simulink model "main"  (R2023b)
settings: Solver=ode4  StartTime=0.0  StopTime=100  FixedStep=0.001  RelTol=1e-3  EnableMultiTasking=on
PreLoadFcn:
  | UserInputs;
libraries: uavalgslib x1, simulink x1
settings Model: DataDictionary=topLevel.sldd  Creator=luke  LastModifiedBy=luke
settings DebuggingCC: InheritedTsInSrcMsg=none
settings ModelReferenceCC: EnableRefExpFcnMdlSchedulingChecks=on  PropagateSignalLabelsOutOfModel=off

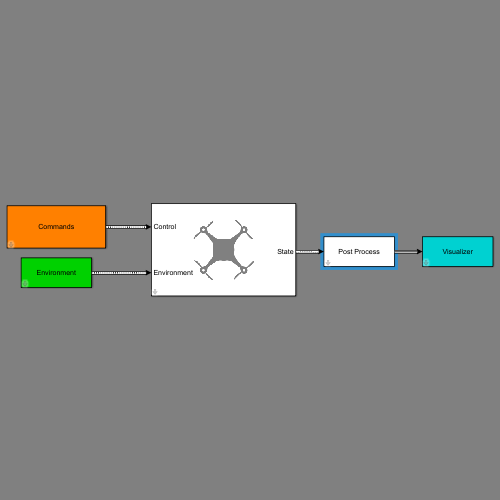
[thumbnail: Simulink's stored preview of the top-level diagram]
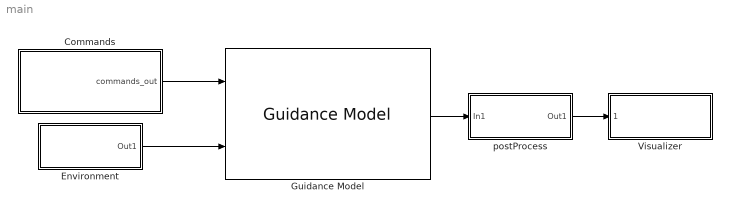
== system main ==
  Commands : Subsystem
      mask Display: disp('Commands');
  Environment : Subsystem
      mask Display: disp('Environment');
  Guidance Model : uavalgslib/Guidance Model  ModelType=MultirotorGuidance  SpecifiedDataType=double  SimulateUsing=Interpreted execution  InitialWorldPositionMultirotor=[0; 0; 200]  InitialWorldVelocityMultirotor=[10; 0; 0]  InitialEulerZYXMultirotor=[0; 0.1; 0]  InitialBodyAngularRateRPYMultirotor=[0; 0; 0]  InitialThrustMultirotor=0  InitialNorthFixedWing=0  InitialEastFixedWing=0  InitialHeightFixedWing=10  InitialAirSpeedFixedWing=0  InitialHeadingAngleFixedWing=0  InitialFlightPathAngleFixedWing=0  InitialRollAngleFixedWing=0  InitialRollAngleRateFixedWing=0  PDRollMultirotor=[3402.97,116.67]  PDPitchMultirotor=[3402.97, 116.67]  PYawRateMultirotor=1950  PThrustMultirotor=3900  MassMultirotor=0.1  PHeightFixedWing=3.9  PHeadingAngleFixedWing=3.9  PFlightPathAngleFixedWing=39  PDRollFixedWing=[3402.97, 116.67]  PAirSpeedFixedWing=1  FlightPathAngleLimitsFixedWing=[-pi/2, pi/2]  StateBusName='StateBus'  ControlBusName='ControlBus'  EnvironmentBusName='EnvironmentBus'  DataType=double
  Visualizer : Subsystem  ReferencedSubsystem=Visualizer
  postProcess : Subsystem
      mask Display: disp("Post Process");
  wires:
  Commands/1(commands_out) -> Guidance Model/1
  Guidance Model/1 -> postProcess/1(In1)
  Environment/1(Out1) -> Guidance Model/2
  postProcess/1(Out1) -> Visualizer/1

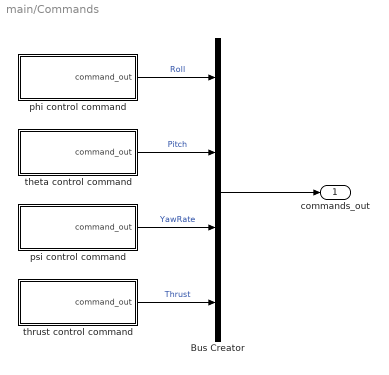
== system main/Commands ==
  Bus Creator : BusCreator  Inputs=4  OutDataTypeStr=Bus: ControlBus  NonVirtualBus=on
      settings: InheritFromInputs=off
  phi control command : Subsystem  Variant=on
      mask Display: disp('\phi Control Command', 'Texmode', 'on');
  psi control command : Subsystem  Variant=on
      mask Display: disp('\psi Control Command', 'Texmode', 'on');
  theta control command : Subsystem  Variant=on
      mask Display: disp('\theta Control Command', 'Texmode', 'on');
  thrust control command : Subsystem  Variant=on
      mask Display: disp('Thrust Control Command');
  commands_out : Outport  OutDataTypeStr=Bus: ControlBus
  wires:
  Bus Creator/1 -> commands_out/1
  theta control command/1(command_out) -> Bus Creator/2  "Pitch"
  phi control command/1(command_out) -> Bus Creator/1  "Roll"
  psi control command/1(command_out) -> Bus Creator/3  "YawRate"
  thrust control command/1(command_out) -> Bus Creator/4  "Thrust"

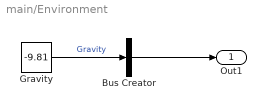
== system main/Environment ==
  Bus Creator : BusCreator  Inputs=1  OutDataTypeStr=Bus: EnvironmentBus  NonVirtualBus=on
      settings: InheritFromInputs=off
  Gravity : Constant  Value=-9.81
  Out1 : Outport  OutDataTypeStr=Bus: EnvironmentBus
  wires:
  Bus Creator/1 -> Out1/1
  Gravity/1 -> Bus Creator/1  "Gravity"

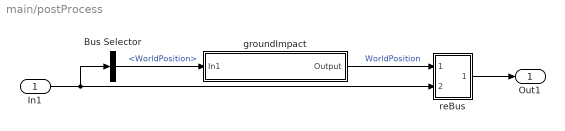
== system main/postProcess ==
  In1 : Inport  OutDataTypeStr=Bus: StateBus
  Bus Selector : BusSelector  OutputSignals=WorldPosition
  groundImpact : Subsystem
      mask Display: disp('Ground Impact');
  reBus : Subsystem
  Out1 : Outport  OutDataTypeStr=Bus: StateBus
  wires:
  reBus/1(Out1) -> Out1/1
  In1/1 -> reBus/2(In1), Bus Selector/1
  groundImpact/1(Output) -> reBus/1(WorldPostion)  "WorldPosition"
  Bus Selector/1 -> groundImpact/1(In1)  "<WorldPosition>"

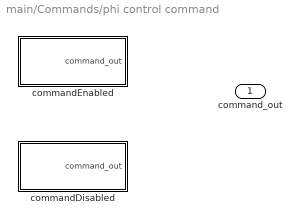
== system main/Commands/phi control command ==
  commandDisabled : Subsystem  VariantControl="userInputs.commands.commandFlags.phiEnable  ==0"
      mask Display: disp('Command Disabled');
  commandEnabled : Subsystem  VariantControl="userInputs.commands.commandFlags.phiEnable  == 1"
      mask Display: disp('Command Enabled');
  command_out : Outport

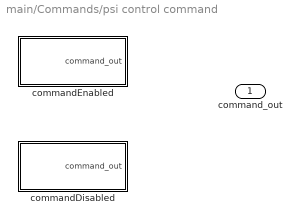
== system main/Commands/psi control command ==
  commandDisabled : Subsystem  VariantControl="userInputs.commands.commandFlags.psiEnable  ==0"
      mask Display: disp('Command Disabled');
  commandEnabled : Subsystem  VariantControl="userInputs.commands.commandFlags.psiEnable  == 1"
      mask Display: disp('Command Enabled');
  command_out : Outport

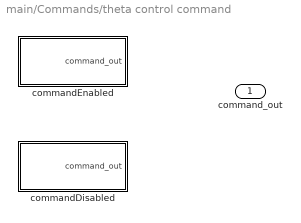
== system main/Commands/theta control command ==
  commandDisabled : Subsystem  VariantControl="userInputs.commands.commandFlags.thetaEnable  ==0"
      mask Display: disp('Command Disabled');
  commandEnabled : Subsystem  VariantControl="userInputs.commands.commandFlags.thetaEnable  == 1"
      mask Display: disp('Command Enabled');
  command_out : Outport

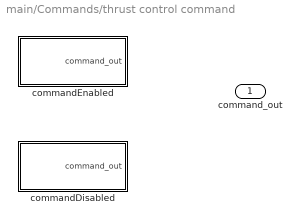
== system main/Commands/thrust control command ==
  commandDisabled : Subsystem  VariantControl="userInputs.commands.commandFlags.thrustEnable  ==0"
      mask Display: disp('Command Disabled');
  commandEnabled : Subsystem  VariantControl="userInputs.commands.commandFlags.thrustEnable  == 1"
      mask Display: disp('Command Enabled');
  command_out : Outport

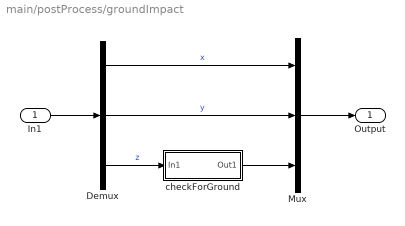
== system main/postProcess/groundImpact ==
  In1 : Inport
  Demux : Demux  Outputs=3
  Mux : Mux  Inputs=3
  checkForGround : Subsystem
  Output : Outport
  wires:
  In1/1 -> Demux/1
  Demux/1 -> Mux/1  "x"
  Demux/2 -> Mux/2  "y"
  Demux/3 -> checkForGround/1(In1)  "z"
  Mux/1 -> Output/1
  checkForGround/1(Out1) -> Mux/3

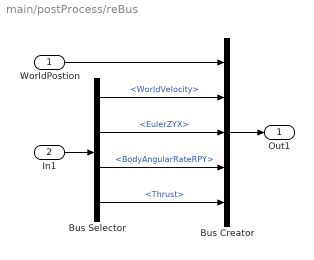
== system main/postProcess/reBus ==
  WorldPostion : Inport
  In1 : Inport  Port=2
  Bus Creator : BusCreator  Inputs=5  OutDataTypeStr=Bus: StateBus
      settings: InheritFromInputs=off
  Bus Selector : BusSelector  OutputSignals=WorldVelocity,EulerZYX,BodyAngularRateRPY,Thrust
  Out1 : Outport  OutDataTypeStr=Bus: StateBus
  wires:
  In1/1 -> Bus Selector/1
  Bus Creator/1 -> Out1/1
  Bus Selector/4 -> Bus Creator/5  "<Thrust>"
  Bus Selector/3 -> Bus Creator/4  "<BodyAngularRateRPY>"
  Bus Selector/2 -> Bus Creator/3  "<EulerZYX>"
  Bus Selector/1 -> Bus Creator/2  "<WorldVelocity>"
  WorldPostion/1 -> Bus Creator/1

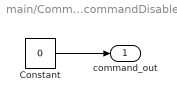
== system main/Commands/phi control command/commandDisabled ==
  Constant : Constant  Value=0
  command_out : Outport
  wires:
  Constant/1 -> command_out/1

== system main/Commands/phi control command/commandEnabled ==
  From Workspace : FromWorkspace  VariableName=userInputs.commands.phi  SampleTime=-1  Interpolate=off  OutputAfterFinalValue=Setting to zero
  command_out : Outport
  wires:
  From Workspace/1 -> command_out/1

== system main/Commands/psi control command/commandDisabled ==
  Constant : Constant  Value=0
  command_out : Outport
  wires:
  Constant/1 -> command_out/1

== system main/Commands/psi control command/commandEnabled ==
  From Workspace : FromWorkspace  VariableName=userInputs.commands.psi  SampleTime=-1  Interpolate=off  OutputAfterFinalValue=Setting to zero
  command_out : Outport
  wires:
  From Workspace/1 -> command_out/1

== system main/Commands/theta control command/commandDisabled ==
  Constant : Constant  Value=0
  command_out : Outport
  wires:
  Constant/1 -> command_out/1

== system main/Commands/theta control command/commandEnabled ==
  From Workspace : FromWorkspace  VariableName=userInputs.commands.theta  SampleTime=-1  Interpolate=off  OutputAfterFinalValue=Setting to zero
  command_out : Outport
  wires:
  From Workspace/1 -> command_out/1

== system main/Commands/thrust control command/commandDisabled ==
  Constant : Constant  Value=0
  command_out : Outport
  wires:
  Constant/1 -> command_out/1

== system main/Commands/thrust control command/commandEnabled ==
  From Workspace : FromWorkspace  VariableName=userInputs.commands.thrust  SampleTime=-1  Interpolate=off  OutputAfterFinalValue=Setting to zero
  command_out : Outport
  wires:
  From Workspace/1 -> command_out/1

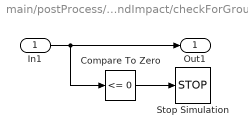
== system main/postProcess/groundImpact/checkForGround ==
  In1 : Inport
  Compare To Zero : simulink/Logic and Bit Operations/Compare To Zero  relop=<=  OutDataTypeStr=boolean
  Stop Simulation : Stop
  Out1 : Outport
  wires:
  In1/1 -> Out1/1, Compare To Zero/1
  Compare To Zero/1 -> Stop Simulation/1
